simulink model "feedback_plant"  (R2019a)
settings: Solver=ode4  StartTime=0.0  StopTime=10.0  FixedStep=0.001  RelTol=1e-3
undefined symbols (not defined in the file): C, g, m, sigbuilder_block
libraries: aerolibanim x2, simulink x1
settings Model: Creator=david  LastModifiedBy=david

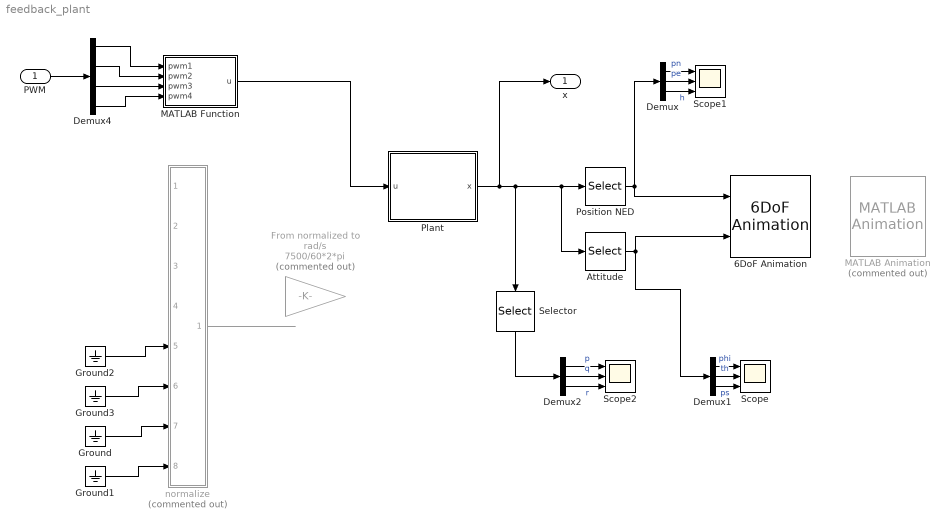
== system feedback_plant ==
  "PWM " : Inport
  6DoF Animation : aerolibanim/6DoF Animation  u1=[0 4000 -2000 2000 -5000 -3000]  u2=0.1  u3=100  u4=[4000 0 -5000]  u5=Fixed position  u6=[2000 500 -3150]  u7=10  u8=off
      settings: SourceProductName=Aerospace Blockset
  Attitude : Selector  InputPortWidth=12  IndexOptions=Index vector (dialog)  Indices=[4:6]  OutputSizes=1
  Demux : Demux  Outputs=3
  Demux1 : Demux  Outputs=3
  Demux2 : Demux  Outputs=3
  Demux4 : Demux
  From normalized to rad/s : Gain  Commented=on  Gain=7500/60*2*pi
  Ground{,1..3} (4 alike) : Ground
  MATLAB Animation : aerolibanim/MATLAB Animation  Tag=Matlab Animation 6 DOF  Commented=on  Vehicles=1  Geometries='astredwedge.mat'  BoundingBoxCoordinates=[-50,50,-50,50,-50,50]  CameraOffset=[-150,-50,0]  CameraViewAngle=3  SampleTime=0.2  FigurePosition=[3.994000e+02,8.740000e+01,5.096000e+02,4.352000e+02]
      settings: SourceProductName=Aerospace Blockset  SourceProductBaseCode=AE
  MATLAB Function : MATLAB Function  TreatAsAtomicUnit=on
  Plant : Subsystem
  Position NED : Selector  InputPortWidth=12  IndexOptions=Index vector (dialog)  Indices=[1:3]  OutputSizes=1
  Scope : Scope  NumInputPorts=3
  Scope1 : Scope  NumInputPorts=3
  Scope2 : Scope  NumInputPorts=3
  Selector : Selector  InputPortWidth=12  IndexOptions=Index vector (dialog)  Indices=[10:12]  OutputSizes=1
  normalize : Subsystem  Commented=on
      mask Display:
      | port_label('input', 1, 'pwm1');
      | port_label('input', 2, 'pwm2');
      | port_label('input', 3, 'pwm3');
      | port_label('input', 4, 'pwm4');
      | port_label('input', 5, 'pwm5');
      | port_label('input', 6, 'pwm6');
      | port_label('input', 7, 'pwm7');
      | port_label('input', 8, 'pwm8');
  x : Outport
  wires:
  Demux1/2 -> Scope/2  "th"
  Demux/3 -> Scope1/3  "h"
  Demux/1 -> Scope1/1  "pn"
  Demux/2 -> Scope1/2  "pe"
  Demux1/3 -> Scope/3  "ps"
  Plant/1(x) -> x/1, Attitude/1, Position NED/1, Selector/1
  Attitude/1 -> 6DoF Animation/2, Demux1/1
  Position NED/1 -> 6DoF Animation/1, Demux/1
  Demux1/1 -> Scope/1  "phi"
  "PWM "/1 -> Demux4/1
  Demux4/2 -> MATLAB Function/2(pwm2)
  Demux4/4 -> MATLAB Function/4(pwm4)
  Ground1/1 -> normalize/8(pwm8)
  Ground3/1 -> normalize/6(pwm6)
  Demux4/1 -> MATLAB Function/1(pwm1)
  Ground2/1 -> normalize/5(pwm5)
  Demux4/3 -> MATLAB Function/3(pwm3)
  Ground/1 -> normalize/7(pwm7)
  normalize/1(normalized_signals) -> ?
  MATLAB Function/1(u) -> Plant/1("u ")
  Demux2/1 -> Scope2/1  "p"
  Demux2/2 -> Scope2/2  "q"
  Demux2/3 -> Scope2/3  "r"
  Selector/1 -> Demux2/1

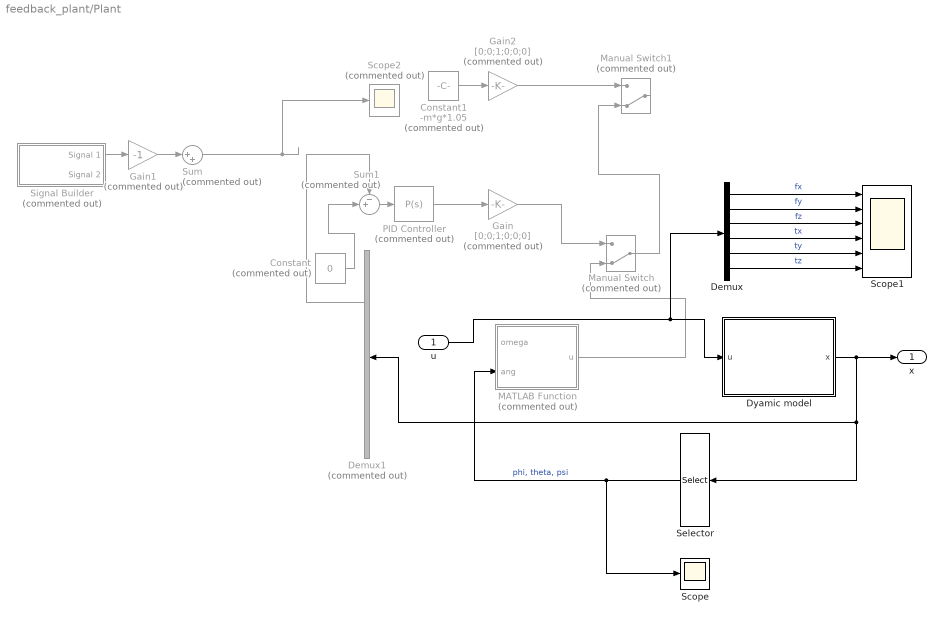
== system feedback_plant/Plant ==
  "u " : Inport
  Constant : Constant  Commented=on  Value=0
  Constant1 : Constant  Commented=on  Value=-m*g*1.05
  Demux : Demux  Outputs=6
  Demux1 : Demux  Commented=on  Outputs=12
  Dyamic model : Subsystem
  Gain : Gain  Commented=on  Gain=[0;0;1;0;0;0]
  Gain1 : Gain  Commented=on  Gain=-1
  Gain2 : Gain  Commented=on  Gain=[0;0;1;0;0;0]
  MATLAB Function : MATLAB Function  Commented=on  TreatAsAtomicUnit=on
  Manual Switch : ManualSwitch  Commented=on  CurrentSetting=0
  Manual Switch1 : ManualSwitch  Commented=on  CurrentSetting=0
  PID Controller : simulink/Continuous/PID Controller  Commented=on  Controller=P  Form=Parallel  TimeDomain=Continuous-time  SampleTime=-1  IntegratorMethod=Forward Euler  FilterMethod=Forward Euler  ControllerParametersSource=internal  P=2  I=1  D=0  UseFilter=on  N=100  TunerSelectOption=Transfer Function Based (PID Tuner App)  InitialConditionSource=internal  InitialConditionForIntegrator=0  InitialConditionForFilter=0  DifferentiatorICPrevScaledInput=0  ExternalReset=none  TrackingMode=off  Kt=1  LimitOutput=off  UpperSaturationLimit=inf  LowerSaturationLimit=-inf  LinearizeAsGain=on  AntiWindupMode=none  Kb=1  POutMin=[]  POutMax=[]  IOutMin=[]  IOutMax=[]  DOutMin=[]  DOutMax=[]  NOutMin=[]  NOutMax=[]  SumOutMin=[]  SumOutMax=[]  SaturationOutMin=[]  SaturationOutMax=[]  PParamMin=[]  PParamMax=[]  IParamMin=[]  IParamMax=[]  DParamMin=[]  DParamMax=[]  NParamMin=[]  NParamMax=[]  KbParamMin=[]  KbParamMax=[]  KtParamMin=[]  KtParamMax=[]  KbOutMin=[]  KbOutMax=[]  KtOutMin=[]  KtOutMax=[]  IntegratorOutMin=[]  IntegratorOutMax=[]  FilterOutMin=[]  FilterOutMax=[]  SumI1OutMin=[]  SumI1OutMax=[]  SumI2OutMin=[]  SumI2OutMax=[]  SumI3OutMin=[]  SumI3OutMax=[]  SumI4OutMin=[]  SumI4OutMax=[]  SumDOutMin=[]  SumDOutMax=[]  DifferentiatorOutMin=[]  DifferentiatorOutMax=[]  FilterDiffOutCoefMin=[]  FilterDiffOutCoefMax=[]  ReciprocalOutMin=[]  ReciprocalOutMax=[]  SumDenOutMin=[]  SumDenOutMax=[]  SumNumOutMin=[]  SumNumOutMax=[]  DivideOutMin=[]  DivideOutMax=[]  IntegratorContinuousStateAttributes=''  IntegratorStateMustResolveToSignalObject=off  IntegratorRTWStateStorageClass=Auto  FilterContinuousStateAttributes=''  FilterStateMustResolveToSignalObject=off  FilterRTWStateStorageClass=Auto  ParallelPVariant=InternalParameters  IdealPVariant=Disabled  IVariant=Disabled  DVariant=Disabled  IntegratorVariant=Disabled  SatVariant=Disabled  AWVariant=Disabled  PCopyVariant=Disabled  TRVariant=Disabled  FdbkBlocksVariant=Forward  IdealPFdbkVariant=Disabled  SatFdbkVariant=Disabled  DerivativeFilterVariant=Disabled  NVariant=Disabled  NCopyVariant=Disabled_SignalSpec  FilterICVariant=Disabled  IntegratorICVariant=Disabled  ExternalResetVariant=Disabled  TRSumVariant=Passthrough  SumFdbkVariant=Disabled  SumVariant=Passthrough_P
  Scope : Scope
  Scope1 : Scope  NumInputPorts=6
  Scope2 : Scope  Commented=on
  Selector : Selector  InputPortWidth=12  IndexOptions=Index vector (dialog)  Indices=[4:6]  OutputSizes=1
  Signal Builder : Subsystem  Tag=STV Subsys  Commented=on  LoadFcn=sigbuilder_block('load');  StartFcn=sigbuilder_block('start');  StopFcn=sigbuilder_block('stop');  ClipboardFcn=sigbuilder_block('clipboard');  mask(Sigbuilder block){tuvar=[0:10]}
      mask help: Simulink:masks:SigbuilderBlock_MD
      mask init:
      | if ~strcmp(get_param(bdroot(gcbh),'SimulationStatus'),'stopped') tuvar = sigbuilder_block('maskInit'); end
      settings: CopyFcn=sigbuilder_block('copy');  DeleteFcn=sigbuilder_block('delete');  ModelCloseFcn=sigbuilder_block('modelClose');  PreSaveFcn=sigbuilder_block('preSave');  PauseFcn=sigbuilder_block('pause');  ContinueFcn=sigbuilder_block('continue');  NameChangeFcn=sigbuilder_block('namechange');  OpenFcn=sigbuilder_block('open',[5.4 30 1141.2 522.6 ]);  CloseFcn=sigbuilder_block('close');
      mask Display: plot(0, 0, 100, 100,[2, 2, 32, 32, 2], [68, 8, 8, 68, 68],[32, 2], [38, 38], [32, 19, 2],[53, 60, 44], [32, 17, 17, 2],[16, 16, 31, 31]);txt = getActiveGroup(gcbh);text(2, 100, txt,'verticalAlignment', 'top');
  Sum : Sum  Commented=on  Inputs=|++
  Sum1 : Sum  Commented=on  Inputs=-+|
  x : Outport
  wires:
  MATLAB Function/1(u) -> Manual Switch/2
  Dyamic model/1(x) -> x/1, Demux1/1, Selector/1
  Selector/1 -> Scope/1, MATLAB Function/2(ang)  "phi, theta, psi"
  Demux/1 -> Scope1/1  "fx"
  Demux/2 -> Scope1/2  "fy"
  Demux/3 -> Scope1/3  "fz"
  Demux/4 -> Scope1/4  "tx"
  Demux/5 -> Scope1/5  "ty"
  Demux/6 -> Scope1/6  "tz"
  Signal Builder/1(Signal 1) -> Gain1/1
  Gain/1 -> Manual Switch/1
  PID Controller/1 -> Gain/1
  Sum1/1 -> PID Controller/1
  Sum/1 -> Scope2/1
  Gain1/1 -> Sum/1
  Constant/1 -> Sum1/2
  Demux1/3 -> Sum1/1
  Manual Switch/1 -> Manual Switch1/2
  Constant1/1 -> Gain2/1
  "u "/1 -> Demux/1, Dyamic model/1(u)
  Gain2/1 -> Manual Switch1/1

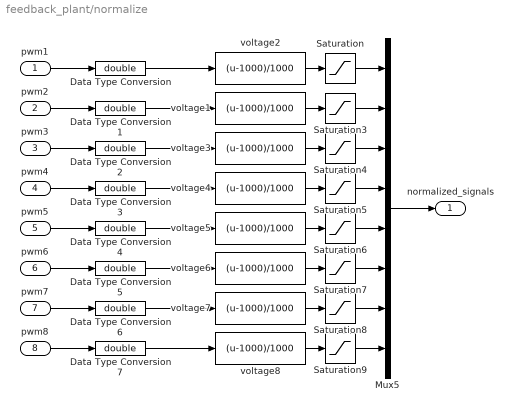
== system feedback_plant/normalize ==
  pwm1 : Inport
  pwm2 : Inport  Port=2
  pwm3 : Inport  Port=3
  pwm4 : Inport  Port=4
  pwm5 : Inport  Port=5
  pwm6 : Inport  Port=6
  pwm7 : Inport  Port=7
  pwm8 : Inport  Port=8
  Data Type Conversion{,1..7} (8 alike) : DataTypeConversion  OutDataTypeStr=double
  Mux5 : Mux  Inputs=8
  Saturation{,3..9} (8 alike) : Saturate  UpperLimit=1  LowerLimit=0
  voltage{1..8} (8 alike) : Fcn  Expr=(u-1000)/1000
  normalized_signals : Outport
  wires:
  voltage1/1 -> Saturation3/1
  Saturation3/1 -> Mux5/2
  Saturation/1 -> Mux5/1
  Saturation6/1 -> Mux5/5
  voltage5/1 -> Saturation6/1
  pwm2/1 -> Data Type Conversion1/1
  pwm5/1 -> Data Type Conversion4/1
  pwm4/1 -> Data Type Conversion3/1
  pwm8/1 -> Data Type Conversion7/1
  pwm6/1 -> Data Type Conversion5/1
  pwm7/1 -> Data Type Conversion6/1
  Saturation4/1 -> Mux5/3
  voltage3/1 -> Saturation4/1
  pwm1/1 -> Data Type Conversion/1
  Mux5/1 -> normalized_signals/1
  pwm3/1 -> Data Type Conversion2/1
  Saturation9/1 -> Mux5/8
  voltage8/1 -> Saturation9/1
  Saturation8/1 -> Mux5/7
  voltage7/1 -> Saturation8/1
  voltage2/1 -> Saturation/1
  voltage4/1 -> Saturation5/1
  voltage6/1 -> Saturation7/1
  Saturation7/1 -> Mux5/6
  Saturation5/1 -> Mux5/4
  Data Type Conversion/1 -> voltage2/1
  Data Type Conversion1/1 -> voltage1/1
  Data Type Conversion2/1 -> voltage3/1
  Data Type Conversion3/1 -> voltage4/1
  Data Type Conversion4/1 -> voltage5/1
  Data Type Conversion5/1 -> voltage6/1
  Data Type Conversion6/1 -> voltage7/1
  Data Type Conversion7/1 -> voltage8/1

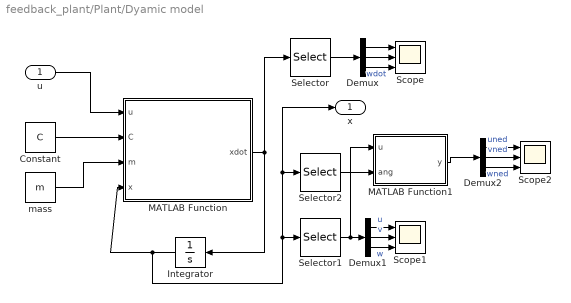
== system feedback_plant/Plant/Dyamic model ==
  u : Inport
  Constant : Constant  Value=C
  Demux : Demux  Outputs=3
  Demux1 : Demux  Outputs=3
  Demux2 : Demux  Outputs=3
  Integrator : Integrator
  MATLAB Function : MATLAB Function  TreatAsAtomicUnit=on
  MATLAB Function1 : MATLAB Function  TreatAsAtomicUnit=on
  Scope : Scope  NumInputPorts=3
  Scope1 : Scope  NumInputPorts=3
  Scope2 : Scope  NumInputPorts=3
  Selector : Selector  InputPortWidth=12  IndexOptions=Index vector (dialog)  Indices=[7:9]  OutputSizes=1
  Selector1 : Selector  InputPortWidth=12  IndexOptions=Index vector (dialog)  Indices=[7:9]  OutputSizes=1
  Selector2 : Selector  InputPortWidth=12  IndexOptions=Index vector (dialog)  Indices=[4:6]  OutputSizes=1
  mass : Constant  Value=m
  x : Outport
  wires:
  mass/1 -> MATLAB Function/3(m)
  MATLAB Function/1(xdot) -> Selector/1, Integrator/1
  u/1 -> MATLAB Function/1(u)
  Constant/1 -> MATLAB Function/2(C)
  Demux/1 -> Scope/1
  Demux/2 -> Scope/2
  Demux/3 -> Scope/3  "wdot"
  Selector/1 -> Demux/1
  Integrator/1 -> Selector2/1, x/1, Selector1/1, MATLAB Function/4(x)
  Selector1/1 -> MATLAB Function1/1(u), Demux1/1
  Demux1/1 -> Scope1/1  "u"
  Demux1/2 -> Scope1/2  "v"
  Demux1/3 -> Scope1/3  "w"
  Demux2/1 -> Scope2/1  "uned"
  Demux2/2 -> Scope2/2  "vned"
  Demux2/3 -> Scope2/3  "wned"
  MATLAB Function1/1(y) -> Demux2/1
  Selector2/1 -> MATLAB Function1/2(ang)

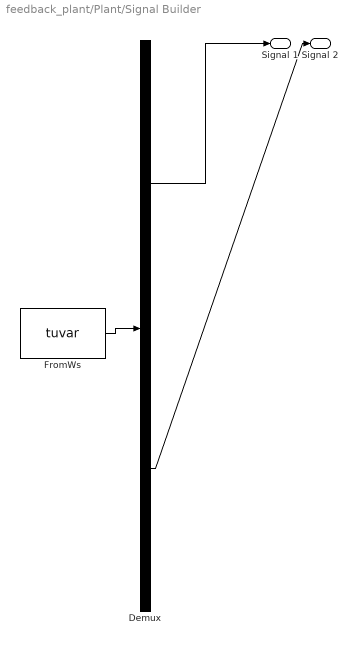
== system feedback_plant/Plant/Signal Builder ==
  Demux : Demux  Tag=STV Demux  Outputs=2
  FromWs : FromWorkspace  Tag=STV FromWs  VariableName=tuvar  SampleTime=0
      SigBuilderData=|
      | common.afterFinalStr = 'Extrapolate'
      | common.sampleTime = 0
      | dataSet.timeRange = [0 30]
      | dataSet.name = 'Group 1'
      | sbobj.Groups.Name = 'Group 1'
      | sbobj.Groups.Signals(1).Name = 'Signal 1'
      | sbobj.Groups.Signals(1).XData = [0 1 1 15 15 30]
      | sbobj.Groups.Signals(1).YData = [0 0 5 5 0 0]
      | sbobj.Groups.Signals(2).Name = 'Signal 2'
      | sbobj.Groups.Signals(2).XData = [0 4 4 6 6 30]
      | sbobj.Groups.Signals(2).YData = [0 0 1 1 0 0]
      | sbobj.Groups.TimeRange = [0 30]
  Signal 1 : Outport  Tag=STV Outport
  Signal 2 : Outport  Tag=STV Outport  Port=2
  wires:
  Demux/1 -> Signal 1/1
  FromWs/1 -> Demux/1
  Demux/2 -> Signal 2/1

== matlab function feedback_plant/Plant/MATLAB Function ==
  data: omega input; u output; ang input
function u = actuator(omega,ang)
% Converts angular speed produced by controller into forces and torques in
% the inertial frame
% global m g Kt Kq l

m = 1.5;
g = 9.81;
Kt = 1.4092e-5;
Kq = 3.9462e-7;
l = 0.2;

u = zeros(6,1);
ph = ang(1);
th = ang(2);
ps = ang(3);

% Changed sign to values related to axis y and z since I'm in NED!!
% u(1:3) = [-sin(th); cos(th)*sin(ps); cos(th)*cos(ps)]*Kt*sum(omega.^2) -...
%     [0; 0; m*g];
u(1:3) = -Kt*sum(omega.^2)*[0; 0; 1];%*[-sin(th); cos(th)*sin(ph); -cos(th)*cos(ph)];
% u(1:3) = [ cos(ps)*sin(th) + cos(th)*sin(ph)*sin(ps)
%             (sin(ps)*sin(th) - cos(ps)*cos(th)*sin(ph))
%             cos(ph)*cos(th) ]*Kt*sum(omega.^2);
u(4) = Kt*l*(omega(3)^2 + omega(2)^2 - omega(1)^2 - omega(4)^2);
u(5) = Kt*l*(omega(1)^2 + omega(3)^2 - omega(2)^2 - omega(4)^2);
u(6) = Kq*(omega(4)^2 + omega(3)^2 - omega(2)^2 - omega(1)^2);

end

== matlab function feedback_plant/Plant/Dyamic model/MATLAB Function ==
  data: u input; C input; m input; x input; xdot output
function xdot = quadrotor_dynamics(u,C,m,x)

ph = x(4);
th = x(5);
ps = x(6);
U = x(7);
V = x(8);
W = x(9);
p = x(10);
q = x(11);
r = x(12);
% Rotation from body to NED
% Rb_ned = [cos(th)*cos(ps), -cos(ph)*sin(ps) + sin(ph)*sin(th)*...
%                 cos(ps), sin(ph)*sin(ps) + cos(ph)*sin(th)*cos(ps)
%             cos(th)*sin(ps), cos(ph)*sin(th)*cos(ps), -sin(ph)*...
%                 cos(ps) + cos(ph)*sin(th)*sin(ps)
%             sin(th), -sin(ph)*cos(th), -cos(ph)*cos(th) ];
        
% Rb_ned = [ cos(ph)*cos(ps), cos(th)*sin(ph), -sin(th)
%             cos(ps)*sin(th)*sin(ps) - cos(ps)*sin(ph), cos(ps)*...
%                 cos(ph) + sin(ph)*sin(th)*sin(ps), cos(th)*sin(ps)
%             sin(ph)*sin(ps) + cos(ph)*cos(ps)*sin(th), cos(ps)*...
%                 sin(ph)*sin(th) - cos(ph)*sin(ps), cos(th)*cos(ps) ];
            
Rb_ned = [ cos(th)*cos(ps), cos(th)*sin(ps), -sin(th)
            -cos(ph)*sin(ps) + sin(ph)*sin(th)*cos(ps), cos(ph)...
                *cos(ps) + sin(ph)*sin(th)*sin(ps), sin(ph)*cos(th)
            sin(ph)*sin(ps) + cos(ph)*sin(th)*cos(ps), -sin(ph)...
            *cos(ps) + cos(ph)*sin(th)*sin(ps), cos(ph)*cos(th) ];
% Rb_ned = zeros(3,3);        
% Rb_ned(1,:) = [cos(ps)*cos(th) -sin(th)*cos(ph)+cos(ps)*sin(th)*sin(ph) sin(ps)*sin(ph)+cos(ps)*cos(ph)*sin(th)];
% Rb_ned(2,:) = [sin(ps)*cos(th) cos(ps)*cos(ph)+sin(ps)*sin(th)*sin(ps) -cos(ps)*sin(ph)+sin(th)*sin(ps)*cos(ph)];
% Rb_ned(3,:) = [-sin(th) cos(th)*sin(ph) cos(th)*cos(ph)];
% Constants linked to Inertia Moments
c1 = C(1);
c2 = C(2);
c3 = C(3);
c4 = C(4);
c5 = C(5);
c6 = C(6);
c7 = C(7);
c8 = C(8);
c9 = C(9);
% Non-linear plant in the form x_dot = f(x) + g(x)*u
f = [ Rb_ned'*x(7:9)
        p + tan(th)*(q*sin(ph) + r*cos(ph))
        q*cos(ph) - r*sin(ph)
        1/cos(th)*(q*sin(ph) + r*cos(ph))
        r*V - q*W - 9.81*sin(th)
        -r*U + p*W + 9.81*sin(ph)*cos(th)
        q*U - p*V + 9.81*cos(ph)*cos(th)
        (c1*r + c2*p)*q
        c5*p*r - c6*(p^2 - r^2) 
        (c8*p - c2*r)*q ];

g = zeros(12,6);
g(7:9,1:3) = diag([1/m,1/m,1/m]);
g(10,4) = c3;
g(10,6) = c4;
g(11,5) = c7;
g(12,4) = c4;
g(12,6) = c9;

xdot = f + g*u;
end

== matlab function feedback_plant/MATLAB Function ==
  data: pwm1 input; u output; pwm2 input; pwm3 input; pwm4 input
function u = fcn(pwm1, pwm2, pwm3, pwm4)

l = 0.2;
P = [1.163247673946401e-05,-0.020227124498192,8.151335788071506];
Q = [2.660432014565793e-07,-4.679737999801719e-04,0.204583957778948];
u = zeros(6,1);
u(3) = -(polyval(P,pwm1) + polyval(P,pwm2) + polyval(P,pwm3) + polyval(P,pwm4));
u(4) = (polyval(P,pwm3) + polyval(P,pwm2) - polyval(P,pwm1) - polyval(P,pwm4))*l;
u(5) = (polyval(P,pwm1) + polyval(P,pwm3) - polyval(P,pwm2) - polyval(P,pwm4))*l;
u(6) = polyval(Q,pwm3) + polyval(Q,pwm4) - polyval(Q,pwm1) - polyval(Q,pwm2);
if u(3) > 0
    u(3) = 0;
end

end

== matlab function feedback_plant/Plant/Dyamic model/MATLAB Function1 ==
  data: u input; y output; ang input
function y = fcn(u,ang)

ph = ang(1);
th = ang(2);
ps = ang(3);

Rb_ned = [ cos(th)*cos(ps), cos(th)*sin(ps), -sin(th)
            -cos(ph)*sin(ps) + sin(ph)*sin(th)*cos(ps), cos(ph)...
                *cos(ps) + sin(ph)*sin(th)*sin(ps), sin(ph)*cos(th)
            sin(ph)*sin(ps) + cos(ph)*sin(th)*cos(ps), -sin(ph)...
            *cos(ps) + cos(ph)*sin(th)*sin(ps), cos(ph)*cos(th) ];
        
y = Rb_ned'*u;

end
